simulink model "testEmplanner_cs_old"  (R2021b)
settings: Solver=ode5  StartTime=0.0  StopTime=60  FixedStep=1/1000  RelTol=1e-3
PreLoadFcn:
  | mbxruntime.callbacks.PreLoadFcn(bdroot);
PostLoadFcn:
  | mbxruntime.callbacks.PostLoadFcn(bdroot);
InitFcn:
  | mbxruntime.callbacks.InitFcn(bdroot);
StartFcn:
  | mbxruntime.callbacks.StartFcn(bdroot);
StopFcn:
  | mbxruntime.callbacks.StopFcn(bdroot);
model workspace (MAT data in the model file):
  mbox_table : object (value not decoded)
  model_closed = 0
  sim_status = 0
values from neighbouring files (symbols this model uses):
  c_factor = 43.75    [emplanner_init.m]
  cf = -175016    [emplanner_init.m]
  cr = -130634    [emplanner_init.m]
  global_path_x = [-1.1448 -0.145417744933 0.852705365581 1.84955224935 2.84511712279 3.83939835808 4.83239585569 5.82411007764 6.81454169183 7.80369144113 8.79156009523 9.77814843293 ... (3001 elements, 3001x1)]    [global_path.mat]
  global_path_y = [14.6488 14.6488 14.6488 14.6488 14.6488 14.6488 14.6488 14.6488 14.6488 14.6488 14.6488 14.6488 ... (3001 elements, 3001x1)]    [global_path.mat]
  KD_PID_distance = 0.0    (= 0)    [emplanner_init.m]
  KD_PID_speed = 0    [emplanner_init.m]
  KI_PID_distance = 0.0    (= 0)    [emplanner_init.m]
  KI_PID_speed = 0    [emplanner_init.m]
  KP_PID_distance = 0.5    [emplanner_init.m]
  KP_PID_speed = 1.8    [emplanner_init.m]
  la = 1.265    [emplanner_init.m]
  lb = 2.947-1.265    (= 1.682)    [emplanner_init.m]
  LQR_K1 = k(:,1)'    [emplanner_init.m]
  LQR_K2 = k(:,2)'    [emplanner_init.m]
  LQR_K3 = k(:,3)'    [emplanner_init.m]
  LQR_K4 = k(:,4)'    [emplanner_init.m]
  m = 2020    [emplanner_init.m]
  rack_displacement = [-39.14 , -37.2 , -35.29 , -33.43 , -31.6 , -29.81 , -28.06 , -26.34 , -24.66 ,      -23.01 , -21.38 , -19.79 , -18.23 , -16.69 , -15.18 , -13.7 , -12.23 , -10.8 , -9.38 , -7.98 ,     -6.61 , -5.25 , -3.91 , -2.59 , -1.29 , 0 , 1.27 , 2.54 , 3.78 , 5.02 , 6.24 , 7.46 , 8.66 ,      9.86 , 11.05 , 12.24 , 13.41 , 14.59 , 15.76 , 16.92 , 18.09 , 19.25 , 20.42 , 21.59 , 22.76 ,      23.93 , 25.11 , 26 ...(+26 chars)    [emplanner_init.m]
  right_wheel_ground = [-70 ,-67.2 , -64.4 , -61.6 , -58.8 , -56 , -53.2 , -50.4 , -47.6 , -44.8 , -42 ,      -39.2 , -36.4 , -33.6 , -30.8 , -28 , -25.2 , -22.4 , -19.6 , -16.8 , -14 , -11.2 , -8.4 , -5.6 ,      -2.8 , 0 , 2.8 , 5.6 , 8.4 , 11.2 , 14 , 16.8 , 19.6 , 22.4 , 25.2 , 28 , 30.8 , 33.6 , 36.4 ,      39.2 , 42 , 44.8 , 47.6 , 50.4 , 53.2 , 56 , 58.8 , 61.6 , 64.4 , 67.2 , 70 ]    [emplanner_init.m]
  vx_break_point = zeros(1,5000)    [emplanner_init.m]
undefined symbols (not defined in the file or in its folder): aubr, DiscIntNeverNeededParam, tablebr, vubr, warningInitialVelocity, x0
libraries: simulink x19, PreScanSimulinkLibrary x17, simulink_extras x6, Solver_SF x1
(part 9 of 14)

== system testEmplanner_cs_old/Audi_A8_Sedan_2/PathFollower_Preview_1/LateralController/SteeringWheelAngle/Sat_Total ==
  In : Inport
  Sat_Limit : Inport  Port=2
  Gain1 : Gain  Gain=-1  SaturateOnIntegerOverflow=on  OutDataTypeStr=Inherit: Same as input  ParamDataTypeStr=Inherit: Same as input
  RelOp_UL : RelationalOperator  RndMeth=Nearest
  RelOp_UL1 : RelationalOperator  Operator=<=  RndMeth=Nearest
  Sum : Sum  Inputs=++|  SaturateOnIntegerOverflow=on
  Switch : Switch  Threshold=0.5  SaturateOnIntegerOverflow=on
  Switch1 : Switch  Threshold=0.5  SaturateOnIntegerOverflow=on
  Sat_Total : Outport
  Sat_Info : Outport  Port=2
  wires:
  Sat_Limit/1 -> Gain1/1, Switch/1, RelOp_UL/2
  RelOp_UL/1 -> Switch/2, Sum/2
  Switch/1 -> RelOp_UL1/1, Switch1/3
  Gain1/1 -> RelOp_UL1/2, Switch1/1
  RelOp_UL1/1 -> Switch1/2, Sum/1
  In/1 -> Switch/3, RelOp_UL/1
  Switch1/1 -> Sat_Total/1
  Sum/1 -> Sat_Info/1

== system testEmplanner_cs_old/Audi_A8_Sedan_2/PathFollower_Preview_1/LongitudinalController/If Desired Velocity ~= 0/PID_AWU ==
  e : Inport
  Derivative Gain : Gain  Gain=D  SaturateOnIntegerOverflow=on  OutDataTypeStr=Inherit: Same as input  ParamDataTypeStr=Inherit: Same as input
  Discrete-Time Integrator : DiscreteIntegrator  gainval=1  SampleTime=CSSampleTime  UpperSaturationLimit=100  LowerSaturationLimit=-100  ICPrevOutput=DiscIntNeverNeededParam  ICPrevScaledInput=DiscIntNeverNeededParam
  Filter : DiscreteIntegrator  gainval=1  SampleTime=CSSampleTime  ICPrevOutput=DiscIntNeverNeededParam  ICPrevScaledInput=DiscIntNeverNeededParam
  Integral Gain : Gain  Gain=I  SaturateOnIntegerOverflow=on  OutDataTypeStr=Inherit: Same as input  ParamDataTypeStr=Inherit: Same as input
  Integral Gain1 : Gain  Gain=LongCtrl_AWU  SaturateOnIntegerOverflow=on  OutDataTypeStr=Inherit: Same as input  ParamDataTypeStr=Inherit: Same as input
  Proportional Gain : Gain  Gain=P  SaturateOnIntegerOverflow=on  OutDataTypeStr=Inherit: Same as input  ParamDataTypeStr=Inherit: Same as input
  Saturation : Saturate  UpperLimit=100  LowerLimit=-100
  Sum : Sum  Inputs=+++  InputSameDT=on  SaturateOnIntegerOverflow=on  OutDataTypeStr=Inherit: Same as first input
  Sum1 : Sum  Inputs=|+-  InputSameDT=on  SaturateOnIntegerOverflow=on  OutDataTypeStr=Inherit: Same as first input
  Sum2 : Sum  Inputs=|++  InputSameDT=on  SaturateOnIntegerOverflow=on  OutDataTypeStr=Inherit: Same as first input
  Sum3 : Sum  Inputs=-+|  InputSameDT=on  SaturateOnIntegerOverflow=on  OutDataTypeStr=Inherit: Same as first input
  u : Outport  InitialOutput=0
  wires:
  Integral Gain1/1 -> Sum2/2
  Sum3/1 -> Integral Gain1/1
  Saturation/1 -> Sum3/2, u/1
  Sum2/1 -> Discrete-Time Integrator/1
  Sum1/1 -> Sum/3, Filter/1
  Filter/1 -> Sum1/2
  Derivative Gain/1 -> Sum1/1
  Sum/1 -> Sum3/1, Saturation/1
  e/1 -> Integral Gain/1, Proportional Gain/1, Derivative Gain/1
  Discrete-Time Integrator/1 -> Sum/2
  Proportional Gain/1 -> Sum/1
  Integral Gain/1 -> Sum2/1

== system testEmplanner_cs_old/Audi_A8_Sedan_2/Trajectories/Traj2State1/Traj2State2/MuxState ==
  x [m] : Inport
  y [m] : Inport  Port=2
  z [m] : Inport  Port=3
  dx [m/s] : Inport  Port=4
  dy [m/s] : Inport  Port=5
  dz [m/s] : Inport  Port=6
  R [rad] : Inport  Port=7
  P [rad] : Inport  Port=8
  Y [rad] : Inport  Port=9
  Mux : Mux  Inputs=9
  state : Outport
  wires:
  z [m]/1 -> Mux/3
  y [m]/1 -> Mux/2
  x [m]/1 -> Mux/1
  Y [rad]/1 -> Mux/9
  P [rad]/1 -> Mux/8
  R [rad]/1 -> Mux/7
  dz [m/s]/1 -> Mux/6
  dy [m/s]/1 -> Mux/5
  dx [m/s]/1 -> Mux/4
  Mux/1 -> state/1

== system testEmplanner_cs_old/Audi_A8_Sedan_2/Trajectories/Traj2State1/Traj2State2/Traj2MuxState_Ext ==
  Traj : Inport
  Terminator{1..9} (9 alike) : Terminator
  demux : Subsystem
  x [m] : Outport
  y [m] : Outport  Port=2
  z [m] : Outport  Port=3
  dx [m/s] : Outport  Port=4
  dy [m/s] : Outport  Port=5
  dz [m/s] : Outport  Port=6
  R [rad] : Outport  Port=7
  P [rad] : Outport  Port=8
  Y [rad] : Outport  Port=9
  wires:
  demux/9(Y) -> Y [rad]/1
  demux/7(R) -> R [rad]/1
  demux/5(vely) -> dy [m/s]/1
  demux/4(velx) -> dx [m/s]/1
  demux/10(velR) -> Terminator4/1
  demux/11(velP) -> Terminator5/1
  demux/12(velY) -> Terminator1/1
  demux/13(accx) -> Terminator8/1
  demux/14(accy) -> Terminator9/1
  demux/15(accz) -> Terminator7/1
  demux/18(accY) -> Terminator2/1
  demux/16(accR) -> Terminator3/1
  demux/17(accP) -> Terminator6/1
  demux/3(z) -> z [m]/1
  Traj/1 -> demux/1(traj)
  demux/6(velz) -> dz [m/s]/1
  demux/1(x) -> x [m]/1
  demux/2(y) -> y [m]/1
  demux/8(P) -> P [rad]/1

== system testEmplanner_cs_old/Audi_A8_Sedan_2/Dynamics_Simple/Chassis/Bicycle_model_[XYZ]/X_Motion/Air&RoadResistance ==
  vx_[ms-1] : Inport
  Gain : Gain  Gain=1/p.Rw
  Road & Aerodyn Resistances : Fcn  Expr=p.Rroad + p.Rair*u^2
  Saturation1 : Saturate  UpperLimit=5/15  LowerLimit=-5/15
  Sign : Signum
  "[ms-1] 2 [rads-1]" : Gain  Gain=1/p.Rw  SaturateOnIntegerOverflow=on  OutDataTypeStr=Inherit: Same as input  ParamDataTypeStr=Inherit: Same as input
  signed load1 : Product  InputSameDT=on  SaturateOnIntegerOverflow=on  OutDataTypeStr=Inherit: Same as first input
  Resistance_Force : Outport
  wires:
  signed load1/1 -> Resistance_Force/1  "F_[N]"
  vx_[ms-1]/1 -> Road & Aerodyn Resistances/1, "[ms-1] 2 [rads-1]"/1
  Saturation1/1 -> Sign/1
  "[ms-1] 2 [rads-1]"/1 -> Saturation1/1
  Road & Aerodyn Resistances/1 -> Gain/1  "ResistanceTorque_[Nm]"
  Sign/1 -> signed load1/2  "sign"
  Gain/1 -> signed load1/1  "Resistance Force_[N]"

== system testEmplanner_cs_old/Audi_A8_Sedan_2/Dynamics_Simple/Chassis/Bicycle_model_[XYZ]/X_Motion/BrakeSystem ==
  vx_[ms-1] : Inport
  BrakePressure_[bar] : Inport  Port=2
  Gain : Gain  Gain=1/p.Rw
  Saturation : Saturate  UpperLimit=p.PBrakeMax  LowerLimit=0
  Saturation1 : Saturate  UpperLimit=5/15  LowerLimit=-5/15
  Sign : Signum
  "[ms-1] 2 [rads-1]" : Gain  Gain=1/p.Rw  SaturateOnIntegerOverflow=on  OutDataTypeStr=Inherit: Same as input  ParamDataTypeStr=Inherit: Same as input
  braking Q factor : Gain  Gain=p.Qfac  SaturateOnIntegerOverflow=on  OutDataTypeStr=Inherit: Same as input  ParamDataTypeStr=Inherit: Same as input
  signed load1 : Product  InputSameDT=on  SaturateOnIntegerOverflow=on  OutDataTypeStr=Inherit: Same as first input
  BrakeForce : Outport
  BrakeTorqueAbs : Outport  Port=2
  wires:
  braking Q factor/1 -> BrakeTorqueAbs/1, Gain/1
  BrakePressure_[bar]/1 -> Saturation/1
  Saturation/1 -> braking Q factor/1
  vx_[ms-1]/1 -> "[ms-1] 2 [rads-1]"/1
  Saturation1/1 -> Sign/1
  "[ms-1] 2 [rads-1]"/1 -> Saturation1/1
  Sign/1 -> signed load1/2  "sign"
  signed load1/1 -> BrakeForce/1
  Gain/1 -> signed load1/1

== system testEmplanner_cs_old/Audi_A8_Sedan_2/Dynamics_Simple/Chassis/Bicycle_model_[XYZ]/X_Motion/Configurable Subsystem ==
  In1 : Inport
  In2 : Inport  Port=2
  In3 : Inport  Port=3
  Integrator : Integrator  ExternalReset=level  InitialConditionSource=external
  Out1 : Outport
  wires:
  In1/1 -> Integrator/1
  In2/1 -> Integrator/2
  In3/1 -> Integrator/3
  Integrator/1 -> Out1/1

== system testEmplanner_cs_old/Audi_A8_Sedan_2/Dynamics_Simple/Chassis/Bicycle_model_[XYZ]/X_Motion/Configurable Subsystem1 ==
  In1 : Inport
  Torsional damping : TransferFcn  Denominator=[0.1 1]
  Out1 : Outport
  wires:
  In1/1 -> Torsional damping/1
  Torsional damping/1 -> Out1/1

== system testEmplanner_cs_old/Audi_A8_Sedan_2/Dynamics_Simple/Chassis/Bicycle_model_[XYZ]/X_Motion/Max RPM and zero- velocity detection ==
  note: Set to zero after infinite small time-step
  note: Zero velocity detection
  ax : Inport
  Drive Torque : Inport  Port=2
  Brake Torque : Inport  Port=3
  v0 : Inport  Port=4
  vx : Inport  Port=5
  Abs : Abs
  Abs1 : Abs
  Compare To Zero : simulink/Logic and Bit Operations/Compare To Zero  relop=<=  OutDataTypeStr=boolean  ZeroCross=off
  Compare To Zero1 : simulink/Logic and Bit Operations/Compare To Zero  relop=>=  OutDataTypeStr=boolean  ZeroCross=off
  Compare To Zero2 : simulink/Logic and Bit Operations/Compare To Zero  relop=>=  OutDataTypeStr=boolean  ZeroCross=off
  Compare To Zero3 : simulink/Logic and Bit Operations/Compare To Zero  relop=<=  OutDataTypeStr=boolean  ZeroCross=off
  Configurable Subsystem : Subsystem  BlockChoice=Step  mask{ComputationMode=ComputationMode}
      mask prompts: ComputationMode "Compuation mode:"
      mask init:
      | SetComputationMode(gcb,ComputationMode);
      settings: AttributesFormatString=%<BlockChoice>  OpenFcn=BringToFront(gcb);  MemberBlocks=Discrete Step,Step
      settings: TemplateBlock=|
      | PreScanSimulinkLibrary/Configurable Subsystems/Step Function/Configurable
      | Subsystem
  Constant : Constant
  Constant1 : Constant
  Logical Operator : Logic  AllPortsSameDT=off  OutDataTypeStr=boolean
  Logical Operator1 : Logic  AllPortsSameDT=off  OutDataTypeStr=boolean
  Logical Operator2 : Logic  Operator=NOT  AllPortsSameDT=off  OutDataTypeStr=boolean
  Logical Operator3 : Logic  AllPortsSameDT=off  OutDataTypeStr=boolean
  Logical Operator4 : Logic  Operator=OR  AllPortsSameDT=off  OutDataTypeStr=boolean
  Memory : Memory
  Memory1 : Memory
  Memory2 : Memory
  Product : Product  RndMeth=Zero
  Relational Operator : RelationalOperator  Operator=<  OutDataTypeStr=boolean  RndMeth=Nearest
  SR-Memory : Subsystem
  Sum : Sum  Inputs=|-+
  Switch : Switch  Criteria=u2 ~= 0  Threshold=0.5
  ax is 0 : Constant  Value=0
  ax_out : Outport
  vx_reset : Outport  Port=2
  x0 : Outport  Port=3
  wires:
  Logical Operator4/1 -> Logical Operator1/1
  vx/1 -> Compare To Zero/1, Compare To Zero2/1, Memory2/1, Memory/1  "vx"
  Memory2/1 -> Compare To Zero3/1
  Compare To Zero2/1 -> Logical Operator3/1
  Compare To Zero3/1 -> Logical Operator3/2
  Logical Operator3/1 -> Logical Operator4/2  "zero-crossing backward"
  Memory/1 -> Compare To Zero1/1
  Compare To Zero/1 -> Logical Operator/1
  Compare To Zero1/1 -> Logical Operator/2
  Logical Operator/1 -> Logical Operator4/1  "zero-crossing forward"
  Abs/1 -> Relational Operator/1
  Abs1/1 -> Relational Operator/2
  Drive Torque/1 -> Abs/1
  Brake Torque/1 -> Abs1/1
  Relational Operator/1 -> Logical Operator1/2, Logical Operator2/1
  Logical Operator1/1 -> SR-Memory/2(Set)
  Constant/1 -> SR-Memory/1(Signal)
  Logical Operator2/1 -> SR-Memory/3(Reset)
  SR-Memory/1(Out) -> Sum/1, Memory1/1
  Switch/1 -> ax_out/1
  Sum/1 -> Switch/2
  ax is 0/1 -> Switch/3
  Constant1/1 -> Sum/2
  v0/1 -> Product/1
  Product/1 -> x0/1
  Configurable Subsystem/1(Out1) -> Product/2
  ax/1 -> Switch/1  "ax"
  Memory1/1 -> vx_reset/1  "vx"

== system testEmplanner_cs_old/Audi_A8_Sedan_2/Dynamics_Simple/Chassis/Bicycle_model_[XYZ]/Y & Yaw_Motion/Configurable Subsystem ==
  In1 : Inport
  In2 : Inport  Port=2
  Integrator : Integrator  ExternalReset=level
  Out1 : Outport
  wires:
  In1/1 -> Integrator/1
  In2/1 -> Integrator/2
  Integrator/1 -> Out1/1

== system testEmplanner_cs_old/Audi_A8_Sedan_2/Dynamics_Simple/Chassis/Bicycle_model_[XYZ]/Y & Yaw_Motion/Configurable Subsystem1 ==
  In1 : Inport
  Integrator : Integrator
  Out1 : Outport
  wires:
  In1/1 -> Integrator/1
  Integrator/1 -> Out1/1

== system testEmplanner_cs_old/Audi_A8_Sedan_2/Dynamics_Simple/Chassis/Bicycle_model_[XYZ]/Y & Yaw_Motion/Configurable Subsystem2 ==
  In1 : Inport
  In2 : Inport  Port=2
  Integrator : Integrator  ExternalReset=level
  Out1 : Outport
  wires:
  In1/1 -> Integrator/1
  In2/1 -> Integrator/2
  Integrator/1 -> Out1/1

== system testEmplanner_cs_old/Audi_A8_Sedan_2/Dynamics_Simple/Chassis/Bicycle_model_[XYZ]/Z, Pitch_Motion & Roll_Motion/Configurable Subsystem ==
  In1 : Inport
  Integrator : Integrator  LimitOutput=on  UpperSaturationLimit=5*pi/180  LowerSaturationLimit=-5*pi/180
  Out1 : Outport
  wires:
  In1/1 -> Integrator/1
  Integrator/1 -> Out1/1

== system testEmplanner_cs_old/Audi_A8_Sedan_2/Dynamics_Simple/Chassis/Bicycle_model_[XYZ]/Z, Pitch_Motion & Roll_Motion/Configurable Subsystem1 ==
  In1 : Inport
  Integrator : Integrator
  Out1 : Outport
  wires:
  In1/1 -> Integrator/1
  Integrator/1 -> Out1/1

== system testEmplanner_cs_old/Audi_A8_Sedan_2/Dynamics_Simple/Chassis/Bicycle_model_[XYZ]/Z, Pitch_Motion & Roll_Motion/Configurable Subsystem2 ==
  In1 : Inport
  Integrator : Integrator
  Out1 : Outport
  wires:
  In1/1 -> Integrator/1
  Integrator/1 -> Out1/1

== system testEmplanner_cs_old/Audi_A8_Sedan_2/Dynamics_Simple/Chassis/Bicycle_model_[XYZ]/Z, Pitch_Motion & Roll_Motion/Configurable Subsystem3 ==
  In1 : Inport
  Integrator : Integrator
  Out1 : Outport
  wires:
  In1/1 -> Integrator/1
  Integrator/1 -> Out1/1

== system testEmplanner_cs_old/Audi_A8_Sedan_2/Dynamics_Simple/Chassis/Bicycle_model_[XYZ]/Z, Pitch_Motion & Roll_Motion/Configurable Subsystem4 ==
  In1 : Inport
  Integrator : Integrator
  Out1 : Outport
  wires:
  In1/1 -> Integrator/1
  Integrator/1 -> Out1/1

== system testEmplanner_cs_old/Audi_A8_Sedan_2/Dynamics_Simple/Chassis/Bicycle_model_[XYZ]/Z, Pitch_Motion & Roll_Motion/Configurable Subsystem5 ==
  In1 : Inport
  Integrator : Integrator
  Out1 : Outport
  wires:
  In1/1 -> Integrator/1
  Integrator/1 -> Out1/1

== system testEmplanner_cs_old/Audi_A8_Sedan_2/Dynamics_Simple/Chassis/Bicycle_model_[XYZ]/Z, Pitch_Motion & Roll_Motion/Configurable Subsystem9 ==
  In1 : Inport
  Derivative : Derivative
  Out1 : Outport
  wires:
  In1/1 -> Derivative/1
  Derivative/1 -> Out1/1

== system testEmplanner_cs_old/Audi_A8_Sedan_2/Dynamics_Simple/Chassis/FrontTyre/AlphaFront/Enabled Subsystem ==
  In : Inport
  Enable : EnablePort  PropagateVarSize=During execution
  AlphaFront : Fcn  Expr=-atan( (u(2)+u(3)*p.a)/u(1) )
  Alpha : Outport  OutputWhenDisabled=reset  InitialOutput=[0]
  wires:
  AlphaFront/1 -> Alpha/1
  In/1 -> AlphaFront/1

== system testEmplanner_cs_old/Audi_A8_Sedan_2/Dynamics_Simple/Chassis/RearTyre/AlphaRear/Enabled Subsystem ==
  In : Inport
  Enable : EnablePort  PropagateVarSize=During execution
  AlphaRear : Fcn  Expr=-atan( (u(2)-u(3)*p.b)/u(1) )
  Alpha : Outport  OutputWhenDisabled=reset  InitialOutput=[0]
  wires:
  AlphaRear/1 -> Alpha/1
  In/1 -> AlphaRear/1

== system testEmplanner_cs_old/Audi_A8_Sedan_2/Trajectories/Traj2State1/Traj2State2/Traj2MuxState_Ext/demux ==
  traj : Inport
  Demux : Demux  Outputs=18
  x : Outport
  y : Outport  Port=2
  z : Outport  Port=3
  velx : Outport  Port=4
  vely : Outport  Port=5
  velz : Outport  Port=6
  R : Outport  Port=7
  P : Outport  Port=8
  Y : Outport  Port=9
  velR : Outport  Port=10
  velP : Outport  Port=11
  velY : Outport  Port=12
  accx : Outport  Port=13
  accy : Outport  Port=14
  accz : Outport  Port=15
  accR : Outport  Port=16
  accP : Outport  Port=17
  accY : Outport  Port=18
  wires:
  Demux/18 -> accY/1
  Demux/17 -> accP/1
  Demux/16 -> accR/1
  Demux/15 -> accz/1
  Demux/14 -> accy/1
  Demux/13 -> accx/1
  Demux/12 -> velY/1
  Demux/11 -> velP/1
  Demux/10 -> velR/1
  Demux/9 -> velz/1
  Demux/8 -> vely/1
  Demux/7 -> velx/1
  Demux/6 -> Y/1
  Demux/5 -> P/1
  traj/1 -> Demux/1
  Demux/4 -> R/1
  Demux/3 -> z/1
  Demux/2 -> y/1
  Demux/1 -> x/1

== system testEmplanner_cs_old/Audi_A8_Sedan_2/Dynamics_Simple/Chassis/Bicycle_model_[XYZ]/X_Motion/Max RPM and zero- velocity detection/Configurable Subsystem ==
  Step : Step  Time=0.0001  Before=1  After=0  SampleTime=0
  Out1 : Outport
  wires:
  Step/1 -> Out1/1

== system testEmplanner_cs_old/Audi_A8_Sedan_2/Dynamics_Simple/Chassis/Bicycle_model_[XYZ]/X_Motion/Max RPM and zero- velocity detection/SR-Memory ==
  Signal : Inport
  Set : Inport  Port=2
  Reset : Inport  Port=3
  Constant : Constant  Value=0
  Detect Rise Positive : simulink/Logic and Bit Operations/Detect Rise Positive  vinit=0  OutDataTypeStr=uint8
  Detect Rise Positive1 : simulink/Logic and Bit Operations/Detect Rise Positive  vinit=0  OutDataTypeStr=uint8
  Manual Switch : ManualSwitch
  Manual Switch1 : ManualSwitch
  Switch : Switch  Criteria=u2 ~= 0
  Switch1 : Switch  Criteria=u2 ~= 0
  Unit Delay : UnitDelay  SampleTime=-1  HasFrameUpgradeWarning=on
  Out : Outport
  wires:
  Constant/1 -> Switch1/1
  Switch/1 -> Switch1/3
  Switch1/1 -> Unit Delay/1, Out/1
  Manual Switch1/1 -> Switch1/2
  Reset/1 -> Manual Switch1/2, Detect Rise Positive1/1
  Detect Rise Positive1/1 -> Manual Switch1/1
  Signal/1 -> Switch/1
  Unit Delay/1 -> Switch/3
  Set/1 -> Detect Rise Positive/1, Manual Switch/2
  Detect Rise Positive/1 -> Manual Switch/1
  Manual Switch/1 -> Switch/2

== matlab function testEmplanner_cs_old/Audi_A8_Sedan_1/decision&planning module/EM Planner1/path decision task/path decision with dynamic planning(dp) ==
  data: obs_s_set input; dp_path_s output; obs_l_set input; plan_start_s input; plan_start_l input; plan_start_dl input; plan_start_dll input; w_cost_collision input; w_cost_smooth_dl input; w_cost_smooth_ddl input; w_cost_smooth_dddl input; w_cost_ref input; row input; col input; sample_s input; sample_l input; dp_path_l output
function [dp_path_s,dp_path_l] = fcn(obs_s_set,obs_l_set,plan_start_s,plan_start_l,plan_start_dl,...
    plan_start_dll,w_cost_collision,w_cost_smooth_dl,w_cost_smooth_ddl,w_cost_smooth_dddl,w_cost_ref,row,col,sample_s,sample_l)
%该函数为路径决策算法动态规划的主函数
% 输入：obs s l set 筛选后的障碍物sl信息
%       plan_start s l dl ddl 规划起点信息
%       w_cost_obs,w_cost_smooth_dl,w_cost_smooth_ddl,w_cost_smooth_dddl,w_cost_ref动态规划代价权重
%       row col 动态规划采样点的行数和列数(row必须是奇数，col必须是6)
%       sample_s,sample_l 采样的s l 长度
% 输出：dp_path_l,dp_path_s 动态规划的路径sl,此路径不包含规划起点  

%动态规划最优的数据结构是结构体矩阵，但是simulink不支持结构体矩阵，所以动态规划算法写的相对难以理解

%声明二维矩阵变量node_cost，node_cost(i,j)表示从起点出发，到行i列j节点的最小代价为node_cost(i,j)
node_cost = ones(row,col)*inf;%初始化为无穷大

%声明二维矩阵变量pre_node_index pre_node_index(i,j)表示从起点到行i列j的节点的最优路径中前一个节点的行号为
%pre_node_index(i,j)
%例：比如一条最优路径为 起点 -> node(1,1) -> node(2,2) -> node(3,3)
%则pre_node_index(3,3) = 2 (最优路径的前一个节点是node(2,2) 取它的行号）
%  pre_node_index(2,2) = 1 (最优路径的前一个节点是node(1,1) 取它的行号）
%  pre_node_index(1,1) = 0 (起点的行号默认是0)

% 其实pre_node_index就是当找到最小代价的路径后从终点到起点反向选择出最优路径的
%如果用结构体矩阵完全没有必要弄得这么麻烦，但是simulink不支持
pre_node_index = zeros(row,col);%初始化，所有节点的上个最优节点的行号都是0，也就是起点

%先计算从起点到第一列的cost
for i = 1:row
    node_cost(i,1) = CalcStartCost(plan_start_s,plan_start_l,plan_start_dl,...
    plan_start_dll,i,sample_s,sample_l,w_cost_collision,w_cost_smooth_dl,...
    w_cost_smooth_ddl,w_cost_smooth_dddl,w_cost_ref,obs_s_set,obs_l_set,row);
end
% 动态规划主函数，从第二列开始
for j = 2:col
    for i = 1:row
        %计算当前node(i,j)的s l
        cur_node_s = plan_start_s + j * sample_s;
        cur_node_l = ((row + 1)/2 - i) * sample_l;
        %遍历前一列的节点
        for k = 1:row
            %计算前一列节点的s l
            pre_node_s = plan_start_s + (j - 1) * sample_s;
            pre_node_l = ((row + 1)/2 - k) * sample_l;
            cost_neighbour = CalcNeighbourCost(pre_node_s,pre_node_l,cur_node_s,cur_node_l,w_cost_collision,...
    w_cost_smooth_dl,w_cost_smooth_ddl,w_cost_smooth_dddl,w_cost_ref,obs_s_set,obs_l_set);
            %起点到上一个节点的最小代价为node_cost(k,j-1)
            pre_min_cost = node_cost(k,j-1);
            %起点到node_cost(i,j)的最小代价 为node_cost(k,j-1)
            %再加上node(k,j-1)到node(i,j)的代价 (k = 1,2,3,4...row) 中最小的
            cost_temp = pre_min_cost + cost_neighbour;
            if cost_temp < node_cost(i,j)
                node_cost(i,j) = cost_temp;
                %把最优路径上一列节点的行号记录下来
                pre_node_index(i,j) = k;
            end
        end      
    end
end
%找到node_cost最后一列中，cost最小的，记代价最小的行号为index
index = 0;
min_cost = inf;
for i = 1:row
    if node_cost(i,end) < min_cost
        min_cost = node_cost(i,end);
        index = i;
    end
end
%动态规划最优路径初始化
dp_node_list_row = zeros(col,1);
%从后往前逆推
cur_index = index;
for i = 1:col
    %记录cur_index前面节点的行号
    pre_index = pre_node_index(cur_index,end - i + 1);
    %把cur_index放到dp_node_list_row对应的位置
    dp_node_list_row(col - i + 1) = cur_index;
    %再把pre_index 赋给 cur_index 进行下一步递推
    cur_index = pre_index;
end
% 输出初始化，由于事先不知道横纵向的采样列数，因此需要做缓冲
dp_path_s = ones(15,1)*-1;
dp_path_l = ones(15,1)*-1;
for i = 1:col
    dp_path_s(i) = plan_start_s + i * sample_s;
    dp_path_l(i) = ((row + 1) / 2 - dp_node_list_row(i)) * sample_l;
end








end
function cost = CalcNeighbourCost(pre_node_s,pre_node_l,cur_node_s,cur_node_l,w_cost_collision,...
    w_cost_smooth_dl,w_cost_smooth_ddl,w_cost_smooth_dddl,w_cost_ref,obs_s_set,obs_l_set)
% 该函数将计算相邻两个节点之间的cost
  
    start_l = pre_node_l;
    start_dl = 0;
    start_ddl = 0;
    end_l = cur_node_l;
    end_dl = 0;
    end_ddl = 0;
    start_s = pre_node_s;
    end_s = cur_node_s;
    coeff = CalcQuinticCoeffient(start_l,start_dl,start_ddl,end_l,end_dl,end_ddl,start_s,end_s);
    a0 = coeff(1);
    a1 = coeff(2);
    a2 = coeff(3);
    a3 = coeff(4);
    a4 = coeff(5);
    a5 = coeff(6);
    % 取10个点计算cost
    ds = zeros(10,1);
    l = zeros(10,1);
    dl = zeros(10,1);
    ddl = zeros(10,1);
    dddl = zeros(10,1);
    for i = 1:10
        ds(i) = start_s + (i-1)*(end_s - start_s)/10;
    end
    l = a0 * ones(10,1) + a1 * ds + a2 * ds.^2 + a3 * ds.^3 + a4 * ds.^4 + a5 * ds.^5;
    dl = a1 * ones(10,1) + 2 * a2 * ds + 3 * a3 * ds.^2 + 4 * a4 * ds.^3 + 5 * a5 * ds.^4;
    ddl = 2 * a2 * ones(10,1) + 6 * a3 * ds + 12 * a4 * ds.^2 + 20 * a5 * ds.^3;
    dddl = 6 * ones(10,1) * a3 + 24 * a4 * ds + 60 * a5 * ds.^2;
    cost_smooth = w_cost_smooth_dl * (dl' * dl) + w_cost_smooth_ddl * (ddl' * ddl) + w_cost_smooth_dddl * (dddl' * dddl);
    for i = 1:length(ddl)
        if abs(ddl(i))> 0.5 || abs(atan(dl(i))) > 0.4*pi
            cost_smooth = cost_smooth + 1e7;
            break;
        end
    end
    cost_ref = w_cost_ref * (l' * l);
    cost_collision = 0;
    for i = 1:length(obs_s_set)
        if isnan(obs_s_set(i))
            break;
        end
        dlon = ones(10,1) * obs_s_set(i) - ds;
        dlat = ones(10,1) * obs_l_set(i) - l;
        %这里做了非常简化的质点模型，认为障碍物就是一个点
        square_d = dlon.^2 + dlat.^2;
        cost_collision_once = CalcObsCost(w_cost_collision,square_d);
        cost_collision = cost_collision + cost_collision_once;
        % 判断障碍物的左右
        v1 = [ds(end);l(end)] - [ds(1);l(1)];
        v2 = [obs_s_set(i);obs_l_set(i)] - [ds(1);l(1)];
        flag = v1(1)*v2(2) - v1(2)*v2(1);
        if flag < 0 && cost_collision > 0
            cost_collision = cost_collision - 1000;
        end
    end
    
    cost = cost_collision + cost_smooth + cost_ref;


end


function cost = CalcStartCost(begin_s,begin_l,begin_dl,begin_ddl,cur_node_row,sample_s,sample_l,w_cost_collision,...
    w_cost_smooth_dl,w_cost_smooth_ddl,w_cost_smooth_dddl,w_cost_ref,obs_s_set,obs_l_set,row)
    %该函数将计算起点到第一层的cost
    start_l = begin_l;
    start_dl = begin_dl;
    start_ddl = begin_ddl;
    %  . . .
    %  . . . row = 3 中间的行号 = (row + 1) /2 = 2
    %  . . .
    end_l = ((row + 1)/2 - cur_node_row)*sample_l;
    end_dl = 0;
    end_ddl = 0;
    start_s = begin_s;
    end_s = begin_s + sample_s;
    coeff = CalcQuinticCoeffient(start_l,start_dl,start_ddl,end_l,end_dl,end_ddl,start_s,end_s);
    a0 = coeff(1);
    a1 = coeff(2);
    a2 = coeff(3);
    a3 = coeff(4);
    a4 = coeff(5);
    a5 = coeff(6);
    % 取10个点计算cost
    ds = zeros(10,1);
    l = zeros(10,1);
    dl = zeros(10,1);
    ddl = zeros(10,1);
    dddl = zeros(10,1);
    for i = 1:10
        ds(i) = start_s + (i-1)*sample_s/10;
    end
    l = a0 * ones(10,1) + a1 * ds + a2 * ds.^2 + a3 * ds.^3 + a4 * ds.^4 + a5 * ds.^5;
    dl = a1 * ones(10,1) + 2 * a2 * ds + 3 * a3 * ds.^2 + 4 * a4 * ds.^3 + 5 * a5 * ds.^4;
    ddl = 2 * a2 * ones(10,1) + 6 * a3 * ds + 12 * a4 * ds.^2 + 20 * a5 * ds.^3;
    dddl = 6 * ones(10,1) * a3 + 24 * a4 * ds + 60 * a5 * ds.^2;
    cost_smooth = w_cost_smooth_dl * (dl' * dl) + w_cost_smooth_ddl * (ddl' * ddl) + w_cost_smooth_dddl * (dddl' * dddl);
    for i = 1:length(dl)
        if abs(ddl(i))> 0.5 || abs(atan(dl(i))) > 0.4*pi
            cost_smooth = cost_smooth + 1e7;
            break;
        end
    end
    cost_ref = w_cost_ref * (l' * l);
    cost_collision = 0;
    for i = 1:length(obs_s_set)
        if isnan(obs_s_set(i))
            break;
        end
        dlon = ones(10,1) * obs_s_set(i) - ds;
        dlat = ones(10,1) * obs_l_set(i) - l;
        %这里做了非常简化的质点模型，认为障碍物就是一个点
        square_d = dlon.^2 + dlat.^2;
        cost_collision_once = CalcObsCost(w_cost_collision,square_d);
        cost_collision = cost_collision + cost_collision_once;
        % 判断障碍物的左右
        v1 = [ds(end);l(end)] - [ds(1);l(1)];
        v2 = [obs_s_set(i);obs_l_set(i)] - [ds(1);l(1)];
        flag = v1(1)*v2(2) - v1(2)*v2(1);
        if flag < 0 && cost_collision > 0
            cost_collision = cost_collision - 1000;
        end
    end
    
    cost = cost_collision + cost_smooth + cost_ref;
        
end

function obs_cost = CalcObsCost(w_cost_collision,square_d)
%该函数将计算障碍物的距离代价
% 暂定超过4米的cost为0 在4到3米的cost为1000/squard_d,在小于3米的cost为w_cost_collision
%   cost = 0;
%   for i = 1:length(square_d)
%       if (square_d(i) < 16 && square_d(i) > 9) 
%           cost = cost + 500/square_d(i);
%       elseif (square_d(i) <= 9)
%           cost = cost + w_cost_collision;
%       end
%   end
%   obs_cost = cost;
min_d = inf;
for i = 1:length(square_d)
    min_d = min(min_d,square_d(i));
end
    obs_cost = w_cost_collision * 10^(-min_d/3);
end

function coeff = CalcQuinticCoeffient(start_l,start_dl,start_ddl,end_l,end_dl,end_ddl,start_s,end_s)
    % l = a0 + a1*s + a2*s^2 + a3*s^3 + a4*s^4 + a5*s^5
    % l' = a1 + 2 * a2 * s + 3 * a3 * s^2 + 4 * a4 * s^3 + 5 * a5 * s^4
    % l'' = 2 * a2 + 6 * a3 * s + 12 * a4 * s^2 + 20 * a5 * s^3
    start_s2 = start_s * start_s;
    start_s3 = start_s2 * start_s;
    start_s4 = start_s3 * start_s;
    start_s5 = start_s4 * start_s;
    end_s2 = end_s * end_s;
    end_s3 = end_s2 * end_s;
    end_s4 = end_s3 * end_s;
    end_s5 = end_s4 * end_s;
    A = [1,start_s, start_s2,     start_s3,     start_s4,      start_s5;
         0 1,       2 * start_s,  3 * start_s2, 4 * start_s3,  5 * start_s4;
         0 0,       2,            6 * start_s,  12 * start_s2, 20 * start_s3;
         1,end_s, end_s2,     end_s3,     end_s4,      end_s5;
         0,1,     2 * end_s,  3 * end_s2, 4 * end_s3,  5 * end_s4;
         0,0,     2,          6 * end_s,  12 * end_s2, 20 * end_s3;];
    B = [start_l;
         start_dl;
         start_ddl;
         end_l;
         end_dl;
         end_ddl;];
     coeff = A \ B;
    
end

== matlab function testEmplanner_cs_old/Audi_A8_Sedan_1/decision&planning module/EM Planner1/path planning task/generate convex space ==
  data: dp_path_s input; l_min output; dp_path_l input; static_obs_s_set input; static_obs_l_set input; static_obs_length input; static_obs_width input; l_max output
function [l_min,l_max] = fcn(dp_path_s,dp_path_l,static_obs_s_set,static_obs_l_set,static_obs_length,static_obs_width)
    % 该函数将输出每个离散的dp_path_s所对应的l的边界lmin lmax (本质上是质点的凸空间)
    % 输入 动态规划曲线 dp_path_s,dp_path_l
    %      障碍物中心的s l 坐标 static_obs_s,static_obs_l
    %      障碍物的长宽 static_obs_length,static_obs_width 
    % 输出 l_min lmax l 的上下界

    % 输出初始化
    l_min = ones(60,1) * -8;
    l_max = ones(60,1) * 8;
    % 对每个障碍物做遍历
    for i = 1:length(static_obs_s_set)
        if isnan(static_obs_s_set(i))
            break;
        end
        % 计算障碍物的头部和尾部的s
        obs_s_min = static_obs_s_set(i) - static_obs_length/2;
        obs_s_max = static_obs_s_set(i) + static_obs_length/2;
        % 找到dp_path_s 中，与s_head s_end最近的s的编号
        start_index = FindNearIndex(dp_path_s,obs_s_min);
        end_index = FindNearIndex(dp_path_s,obs_s_max);
        path_l = (dp_path_l(start_index) + dp_path_l(end_index))/2;
        if start_index == 1 && end_index == 1
            continue;
        end
        if path_l > static_obs_l_set(i)
            % 意味着决策为向左绕过障碍物
            for j = start_index:end_index
                % l_min(j) 为所有决策为向左绕过障碍物的l边界的最大值
                l_min(j) = max(l_min(j) , static_obs_l_set(i) + static_obs_width/2);
            end
        else
            % 意味着决策为向右绕过障碍物
            for j = start_index:end_index
                % l_max(j) 为所有决策为向右绕过障碍物的l边界的最小值
                l_max(j) = min(l_max(j) , static_obs_l_set(i) - static_obs_width/2);
            end
        end       
    end
end

function y = FindNearIndex(dp_path_s,obs_s)
    % 该函数将找到dp_path_s的所有点中，距离obs_s最近的点的编号
    % 这里要注意obs_s 是在完整的reference line上投影所得到的坐标，所以obs_s可能是负值，也可能会超过dp_path_s最远的长度
    if dp_path_s(1) >= obs_s
        %障碍物在后面
        y = 1;
        return;
    elseif dp_path_s(end) <= obs_s
        y = 60;
        return;
    else
        index = 1;
        while dp_path_s(index) < obs_s
            index = index + 1;
        end
        % 循环退出的条件是dp_path_s(index) >= obs_s 判断一下index 和 index-1哪个离的近
        if dp_path_s(index) - obs_s > obs_s - dp_path_s(index - 1)
            y = index - 1;
        else
            y = index;
        end
    end
end

== matlab function testEmplanner_cs_old/Audi_A8_Sedan_1/decision&planning module/EM Planner1/path planning task/path planning with quadratic programming (qp) ==
  data: l_min input; qp_path_l output; l_max input; w_cost_l input; w_cost_dl input; w_cost_ddl input; w_cost_dddl input; w_cost_centre input; w_cost_end_l input; w_cost_end_dl input; w_cost_end_ddl input; host_d1 input; host_d2 input; host_w input; plan_start_l input; plan_start_dl input; plan_start_ddl input; qp_path_dl output; qp_path_ddl output; dp_path_l_final input
function [qp_path_l,qp_path_dl,qp_path_ddl] = ...
fcn(l_min,l_max,w_cost_l,w_cost_dl,w_cost_ddl,w_cost_dddl,w_cost_centre,w_cost_end_l,w_cost_end_dl,w_cost_end_ddl,...
    host_d1,host_d2,host_w,...
    plan_start_l,plan_start_dl,plan_start_ddl,dp_path_l_final)
% 路径二次规划
% 0.5*x'Hx + f'*x = min
% subject to A*x <= b
%            Aeq*x = beq
%            lb <= x <= ub;
% 输入：l_min l_max 点的凸空间
%       w_cost_l 参考线代价
%       w_cost_dl ddl dddl 光滑性代价
%       w_cost_centre 凸空间中央代价
%       w_cost_end_l dl dd1 终点的状态代价 (希望path的终点状态为(0,0,0))
%       host_d1,d2 host质心到前后轴的距离
%       host_w host的宽度
%       plan_start_l,dl,ddl 规划起点
% 输出 qp_path_l dl ddl 二次规划输出的曲线
coder.extrinsic("quadprog");
% 待优化的变量的数量
n = 60;

% 输出初始化
qp_path_l = zeros(n,1);
qp_path_dl = zeros(n,1);
qp_path_ddl = zeros(n,1);
% H_L H_DL H_DDL H_DDDL Aeq beq A b 初始化
H_L = zeros(3*n, 3*n);
H_DL = zeros(3*n, 3*n);
H_DDL = zeros(3*n, 3*n);
H_DDDL = zeros(n-1, 3*n);
H_CENTRE = zeros(3*n, 3*n);
H_L_END = zeros(3*n, 3*n);
H_DL_END = zeros(3*n, 3*n);
H_DDL_END = zeros(3*n, 3*n);
Aeq = zeros(2*n-2, 3*n);
beq = zeros(2*n-2, 1);
A = zeros(8*n, 3*n);
b = zeros(8*n, 1);
%  期望的终点状态
end_l_desire = 0;
end_dl_desire = 0;
end_ddl_desire = 0;

% Aeq_sub
ds = 1;%纵向间隔
Aeq_sub = [1 ds ds^2/3 -1 0 ds^2/6;
           0 1  ds/2   0 -1 ds/2];
% A_sub;
d1 = host_d1;
d2 = host_d2;
w = host_w;
A_sub = [1  d1 0;
         1  d1 0;
         1 -d2 0;
         1 -d2 0;
        -1 -d1 0;
        -1 -d1 0;
        -1  d2 0;
        -1  d2 0];
% 生成Aeq
for i = 1:n-1
    % 计算分块矩阵左上角的行和列
    row = 2*i - 1;
    col = 3*i - 2;
    Aeq(row:row + 1,col:col + 5) = Aeq_sub;
end
% 生成A
for i = 1:n
    row = 8*i - 7;
    col = 3*i - 2;
    A(row:row + 7,col:col + 2) = A_sub;
end

% 视频里用的找(s(i) - d2,s(i) + d1)的方法过于保守，在这里舍弃掉
% 只要找到四个角点所对应的l_min l_max 即可
% 。。。。。。。。。。。。。。
%    [    .   ]<- 
%    [        ]
% 。。。。。。。。。。。。。
front_index = ceil(d1/ds);
back_index = ceil(d2/ds); % ceil向上取整 ceil(3) = 3 ceil(3.1) = 4
% 生成b
for i = 1:n
    % 左前 右前的index = min(i + front_index,60)
    % 左后 右后的index = max(i - back_index,1)
    index1 = min(i + front_index,n);
    index2 = max(i - back_index,1);
    b(8*i - 7:8*i,1) = [l_max(index1) - w/2;
                        l_max(index1) + w/2;
                        l_max(index2) - w/2;
                        l_max(index2) + w/2;
                       -l_min(index1) + w/2;
                       -l_min(index1) - w/2;
                       -l_min(index2) + w/2;
                       -l_min(index2) - w/2;];
end
%生成 lb ub 主要是对规划起点做约束
lb = ones(3*n,1)*-inf;
ub = ones(3*n,1)*inf;
lb(1) = plan_start_l;
lb(2) = plan_start_dl;
lb(3) = plan_start_ddl;
ub(1) = lb(1);
ub(2) = lb(2);
ub(3) = lb(3);
% for i = 2:n
%     lb(3*i - 1) = - pi/8;
%     ub(3*i - 1) = pi/8;
%     lb(3*i) = -0.1;
%     ub(3*i) = 0.1;
% end
% 生成H_L,H_DL,H_DDL,H_CENTRE
for i = 1:n
    H_L(3*i - 2,3*i - 2) = 1;
    H_DL(3*i - 1,3*i - 1) = 1;
    H_DDL(3*i, 3*i) = 1;
end
H_CENTRE = H_L;
% 生成H_DDDL;
H_dddl_sub = [0 0 1 0 0 -1];
for i = 1:n-1
    row = i;
    col = 3*i - 2;
    H_DDDL(row,col:col + 5) = H_dddl_sub;
end
% 生成H_L_END H_DL_END H_DDL_END
H_L_END(3*n - 2,3*n - 2) = 1;
H_DL_END(3*n - 1,3*n - 1) = 1;
H_DDL_END(3*n,3*n) = 1;
% 生成二次规划的H
H = w_cost_l * (H_L'*H_L) + w_cost_dl * (H_DL'*H_DL) + w_cost_ddl * (H_DDL'*H_DDL)...
   +w_cost_dddl * (H_DDDL'*H_DDDL) + w_cost_centre * (H_CENTRE'*H_CENTRE) + w_cost_end_l * (H_L_END'*H_L_END)...
   +w_cost_end_dl * (H_DL_END'* H_DL_END) + w_cost_ddl * (H_DDL_END'*H_DDL_END);
H = 2 * H;
% 生成f
f = zeros(3*n,1);
 centre_line = 0.5 * (l_min + l_max);
centre_line = dp_path_l_final;
for i = 1:n
    f(3*i - 2) = -2 * centre_line(i);
end

f = w_cost_centre * f;
% 终点要接近end_l dl ddl desire
f(3*n - 2) = f(3*n - 2) -2 * end_l_desire * w_cost_end_l;
f(3*n - 1) = f(3*n - 1) -2 * end_dl_desire * w_cost_end_dl;
f(3*n) = f(3*n) -2 * end_ddl_desire * w_cost_end_ddl;

X = quadprog(H,f,A,b,Aeq,beq,lb,ub);
% 这里没有对曲率做强制约束，并不好
% 可以用 |dl(i+1) - dl(i)|/ds <= kappa_max 近似去约束曲率
for i = 1:n
    qp_path_l(i) = X(3*i - 2);
    qp_path_dl(i) = X(3*i - 1);
    qp_path_ddl(i) = X(3*i);
end

end

== matlab function testEmplanner_cs_old/Audi_A8_Sedan_2/PathFollower_Preview_1/LateralController/CTRL REFERENCES/Find Reference Point (pref0) on Trajectory closest to P0 Point (p0)/eml_find_closest_trajectory_points0 ==
  data: pvp input size=2; Actor_traj_distance output; TrajOffset_x_y_Y input size=3; ActorOffset_Left_Right input; p0 input size=3; Traj_x parameter; Traj_y parameter; Actor_traj_angle output; RefreshCounter parameter
function [Actor_traj_distance,Actor_traj_angle]  = eml_find_closest_trajectory_points0(pvp,TrajOffset_x_y_Y,ActorOffset_Left_Right,p0,Traj_x,Traj_y,RefreshCounter)

[Actor_traj_distance,Actor_traj_angle]  = emlfcn_find_closest_trajectory_points0(pvp,TrajOffset_x_y_Y,ActorOffset_Left_Right,p0,Traj_x,Traj_y,RefreshCounter);

% end function

== matlab function testEmplanner_cs_old/Audi_A8_Sedan_1/decision&planning module/EM Planner1/plot ==
  data: dp_s input; dp_l input; qp_l input; l_min input; l_max input; obs_s_set input; obs_l_set input; start_s input; start_l input; start_dl input
function  fcn(dp_s,dp_l,qp_l,l_min,l_max,obs_s_set,obs_l_set,start_s,start_l,start_dl)
coder.extrinsic("plot","axis","figure","drawnow","cla","fill");

obs_length = 5;
obs_width = 2;
host_l = 6;
host_w = 1.63;
cla;
host_p1_l = start_l + sin(atan(start_dl)) * host_l /2 + host_w/2 * cos(atan(start_dl));
host_p1_s = start_s + cos(atan(start_dl)) * host_l /2 - host_w/2 * sin(atan(start_dl));
host_p2_l = start_l + sin(atan(start_dl)) * host_l /2 - host_w/2 * cos(atan(start_dl));
host_p2_s = start_s + cos(atan(start_dl)) * host_l /2 + host_w/2 * sin(atan(start_dl));
host_p3_l = start_l - sin(atan(start_dl)) * host_l /2 + host_w/2 * cos(atan(start_dl));
host_p3_s = start_s - cos(atan(start_dl)) * host_l /2 - host_w/2 * sin(atan(start_dl));
host_p4_l = start_l - sin(atan(start_dl)) * host_l /2 - host_w/2 * cos(atan(start_dl));
host_p4_s = start_s - cos(atan(start_dl)) * host_l /2 + host_w/2 * sin(atan(start_dl));
host_area_x = [host_p1_s;host_p2_s;host_p4_s;host_p3_s];
host_area_y = [host_p1_l;host_p2_l;host_p4_l;host_p3_l];
fill(host_area_x,host_area_y,[0 1 1]);
hold on
plot(dp_s,dp_l,'r');

plot(dp_s,qp_l,'b');
plot(dp_s,l_min,dp_s,l_max);
axis([-8 70 -10 10]);

for i = 1:length(obs_s_set)
    if isnan(obs_s_set(i))
        break;
    end
    obs_p1_s = obs_s_set(i) + obs_length/2;
    obs_p1_l = obs_l_set(i) + obs_width/2;
    obs_p2_s = obs_s_set(i) + obs_length/2;
    obs_p2_l = obs_l_set(i) - obs_width/2;
    obs_p3_s = obs_s_set(i) - obs_length/2;
    obs_p3_l = obs_l_set(i) + obs_width/2;
    obs_p4_s = obs_s_set(i) - obs_length/2;
    obs_p4_l = obs_l_set(i) - obs_width/2;
    obs_area_s = [obs_p1_s;obs_p2_s;obs_p4_s;obs_p3_s];
    obs_area_l = [obs_p1_l;obs_p2_l;obs_p4_l;obs_p3_l];
    fill(obs_area_s,obs_area_l,[0 0 0]);
end

== matlab function testEmplanner_cs_old/Audi_A8_Sedan_1/decision&planning module/EM Planner1/simple speed qp planning ==
  data: plan_start_s_dot input; s_init output; plan_start_s_dot2 input; s_end input; recommend_T input; s_dot_init output; s_dot2_init output; relative_time_init output
function [s_init,s_dot_init,s_dot2_init,relative_time_init] = fcn(plan_start_s_dot,plan_start_s_dot2,s_end,recommend_T)
%简单速度二次规划
coder.extrinsic("quadprog")
n = 51;
s_init = zeros(n,1);
s_dot_init = zeros(n,1);
s_dot2_init = zeros(n,1);
relative_time_init = zeros(n,1);

Aeq = zeros(3*n,2*n - 2);
beq = zeros(2*n - 2,1);
lb = ones(3*n,1);
ub = lb;
dt = recommend_T/(n-1);
A_sub =[1,0;
        dt,1;
        (1/3)*dt^2,(1/2)*dt;
        -1,0;
        0,-1;
        (1/6)*dt^2,dt/2];
for i = 1:n - 1
    Aeq(3*i-2:3*i+3,2*i-1:2*i) = A_sub;
end

for i = 1:n
   lb(3*i - 2) = -inf;
   lb(3*i - 1) = 0;
   lb(3*i) = -8;
   ub(3*i - 2) = inf;
   ub(3*i - 1) = 50;
   ub(3*i) = 2;
end
lb(1) = 0;
lb(2) = plan_start_s_dot;
lb(3) = plan_start_s_dot2;
ub(1) = lb(1);
ub(2) = lb(2);
ub(3) = lb(3);
lb(3*n - 2) = s_end;
ub(3*n - 2) = s_end;
A3 = zeros(3*n,3*n);
A4 = zeros(3*n,n - 1);
A4_sub =[0;0;1;0;0;-1];
for i = 1:n - 1
   A3(3*i,3*i) = 1;
   A4(3*i-2:3*i+3,i:i) = A4_sub;
end
A3(3*n,3*n) = 1;
H = A3 + 100*(A4*A4');
H = 2*H;
f = zeros(3*n,1);
X = quadprog(H,f,[],[],Aeq',beq,lb,ub);
for i = 1:n
   s_init(i) = X(3*i - 2);
   s_dot_init(i) = X(3*i - 1);
   s_dot2_init(i) = X(3*i);
   relative_time_init(i) = (i - 1)*dt;
end

== matlab function testEmplanner_cs_old/Audi_A8_Sedan_1/decision&planning module/EM Planner1/stitch trajectory ==
  data: trajectory_x input; trajectory_x_final output; trajectory_y input; trajectory_heading input; trajectory_kappa input; trajectory_speed input; trajectory_accel input; trajectory_time input; stitch_x input; stitch_y input; stitch_heading input; stitch_kappa input; stitch_speed input; stitch_accel input; stitch_time input; trajectory_y_final output; trajectory_heading_final output; trajectory_kappa_final output; trajectory_speed_final output; trajectory_accel_final output; trajectory_time_final output
function [trajectory_x_final,trajectory_y_final,trajectory_heading_final,trajectory_kappa_final,...
          trajectory_speed_final,trajectory_accel_final,trajectory_time_final] = fcn(trajectory_x,...
          trajectory_y,trajectory_heading,trajectory_kappa,trajectory_speed,trajectory_accel,trajectory_time,...
          stitch_x,stitch_y,stitch_heading,stitch_kappa,stitch_speed,stitch_accel,stitch_time)
% 轨迹拼接，把stitch trajectory 拼到规划完成的轨迹上
n = 401 + 20;
trajectory_x_final = zeros(n,1);
trajectory_y_final = zeros(n,1);
trajectory_heading_final = zeros(n,1);
trajectory_kappa_final = zeros(n,1);
trajectory_speed_final = zeros(n,1);
trajectory_accel_final = zeros(n,1);
trajectory_time_final = zeros(n,1);

trajectory_x_final = [stitch_x;trajectory_x];
trajectory_y_final = [stitch_y;trajectory_y];
trajectory_heading_final = [stitch_heading;trajectory_heading];
trajectory_kappa_final = [stitch_kappa;trajectory_kappa];
trajectory_speed_final = [stitch_speed;trajectory_speed];
trajectory_accel_final = [stitch_accel;trajectory_accel];
trajectory_time_final = [stitch_time;trajectory_time];

== matlab function testEmplanner_cs_old/Audi_A8_Sedan_1/decision&planning module/EM Planner/Cartesian2Frenet/Cartesian2Frenet ==
  data: x_set input; s_set output; y_set input; frenet_path_x input; frenet_path_y input; proj_x_set input; proj_y_set input; proj_heading_set input; proj_match_point_index_set input; index2s input; l_set output
function [s_set,l_set] = fcn(x_set,y_set,frenet_path_x,frenet_path_y, ...
	proj_x_set,proj_y_set,proj_heading_set,proj_match_point_index_set,index2s)
	%该函数将计算世界坐标系下的x_set,y_set上的点在frenet_path下的坐标s,l 
	%输入： x_set,y_set 待坐标转换的点
	%       frenet_path_x,frenet_path_y frenet坐标轴
	%       proj_x,proj_y heading ,kappa,proj_match_point_index_set 待坐标转换的点的投影点的信息
	% 		index2s frenet_path 的index与s的转换表

	% 由于不知道有多少个点要做坐标转换，所以需要做缓冲
	n = 128;% 最多处理128个点
	%输出做初始化
	s_set = ones(n,1) * nan;
	l_set = ones(n,1) * nan;
	for i = 1: length(x_set)
		if isnan(x_set(i))
			break;
		end
		
		%计算s,写子函数
		s_set(i) = CalcSFromIndex2S(index2s,frenet_path_x,frenet_path_y,proj_x_set(i),proj_y_set(i),proj_match_point_index_set(i));
		
		%第一章第三节说很详细了，查阅第一章第三节
		n_r = [-sin(proj_heading_set(i));cos(proj_heading_set(i))];
		r_h = [x_set(i);y_set(i)];
		r_r = [proj_x_set(i);proj_y_set(i)];
		l_set(i) = (r_h - r_r)' * n_r;
	end

end


function s = CalcSFromIndex2S(index2s,path_x,path_y,proj_x,proj_y,proj_match_point_index)
	%该函数将计算当指定index2s的映射关系后，计算点proj_x,proj_y的弧长
	vector_1 = [proj_x;proj_y] - [path_x(proj_match_point_index);path_y(proj_match_point_index)];
	%这里要考虑的全面一点，因为要考虑到proj_match_point_index有可能在path的起点或者终点
	if (proj_match_point_index < length(path_x))
		vector_2 = [path_x(proj_match_point_index + 1);path_y(proj_match_point_index + 1)] - ...
			[path_x(proj_match_point_index);path_y(proj_match_point_index)];
	else
		vector_2 = [path_x(proj_match_point_index);path_y(proj_match_point_index)] - ...
			[path_x(proj_match_point_index - 1);path_y(proj_match_point_index - 1)];
	end
	
	if  vector_1' * vector_2 > 0 
		s = index2s(proj_match_point_index) + sqrt(vector_1' * vector_1);
	else
		s = index2s(proj_match_point_index) - sqrt(vector_1' * vector_1);
	end
end

== matlab function testEmplanner_cs_old/Audi_A8_Sedan_1/decision&planning module/EM Planner/Cartesian2Frenet/MATLAB Function ==
  data: l_set input; s_dot_set output; vx_set input; vy_set input; proj_heading_set input; proj_kappa_set input; l_dot_set output; dl_set output
function [s_dot_set,l_dot_set,dl_set] = fcn(l_set,vx_set,vy_set,proj_heading_set,proj_kappa_set)
%该函数将计算frenet坐标系下的s_dot,l_dot,dl/ds
n = 128;
%输出初始化
s_dot_set = ones(n,1)*nan;
l_dot_set = ones(n,1)*nan;
dl_set = ones(n,1)*nan;

for i = 1: length(l_set)
	if isnan(l_set(i))
		break;
	end
	v_h = [vx_set(i);vy_set(i)];
	n_r = [-sin(proj_heading_set(i));cos(proj_heading_set(i))];
	t_r = [cos(proj_heading_set(i));sin(proj_heading_set(i))];
	l_dot_set(i) = v_h' * n_r;
	s_dot_set(i) = v_h' * t_r /(1-proj_kappa_set(i)*l_set(i));
	%%%% 向量法做cartesian与frenet的转换要简单，但是也有问题，向量法必须依赖速度加速度
	%l' = l_dot / s_dot但是如果s_dot = 0，此方法就失效了
	if abs(s_dot_set(i)) < 1e-6
		dl_set(i) = 0;
	else
		dl_set(i) = l_dot_set(i) / s_dot_set(i);
	end
end

== matlab function testEmplanner_cs_old/Audi_A8_Sedan_1/decision&planning module/EM Planner/Cartesian2Frenet/MATLAB Function1 ==
  data: ax_set input; s_dot2_set output; ay_set input; proj_heading_set input; proj_kappa_set input; l_set input; s_dot_set input; dl_set input; l_dot2_set output; ddl_set output
function [s_dot2_set,l_dot2_set,ddl_set] = fcn(ax_set,ay_set,proj_heading_set,proj_kappa_set,l_set,s_dot_set,dl_set)
% 由于不知道有多少个点需要做坐标转换，设一个最大值作为缓冲
 n = 128;
% 输出初始化
s_dot2_set = ones(n,1)*nan;
l_dot2_set = ones(n,1)*nan;
ddl_set = ones(n,1)*nan;

for i = 1 : length(l_set)
	if isnan(l_set(i))
		break;
	end
	a_h = [ax_set(i);ay_set(i)];
	n_r = [-sin(proj_heading_set(i));cos(proj_heading_set(i))];
	t_r = [cos(proj_heading_set(i));sin(proj_heading_set(i))];
	%近似认为 dkr/ds为0 简化计算
	l_dot2_set(i) = a_h' *n_r - proj_kappa_set(i) * (1 - proj_kappa_set(i) * l_set(i)) * s_dot_set(i)^2;
	s_dot2_set(i) = (1/ (1 - proj_kappa_set(i) * l_set(i))) * (a_h' * t_r + 2 * proj_kappa_set(i) * dl_set(i) * s_dot_set(i)^2);
	% 要考虑加速度为0的情况
	if abs(s_dot2_set(i)) < 1e-6
		ddl_set(i) = 0;
	else
		ddl_set(i) = (l_dot2_set(i) - dl_set(i)* s_dot2_set(i)) / (s_dot_set(i)^2);
	end
end
